simulink model "unit_delay_demo"  (Simulink 6.3)
settings: Solver=ode45  StartTime=0.0  StopTime=10.0  RelTol=1e-3
settings Model: LastModifiedBy=Ms1

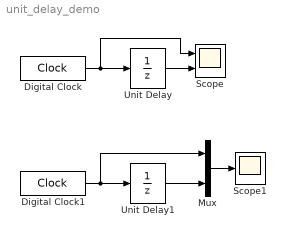
== system unit_delay_demo ==
  Digital Clock : DigitalClock
  Digital Clock1 : DigitalClock
  Mux : Mux  Inputs=2
  Scope : Scope  NumInputPorts=2
      settings: YMin=-5~-5  YMax=5~5
  Scope1 : Scope
  Unit Delay : UnitDelay
  Unit Delay1 : UnitDelay
  wires:
  Digital Clock/1 -> Unit Delay/1, Scope/1
  Unit Delay/1 -> Scope/2
  Digital Clock1/1 -> Unit Delay1/1, Mux/1
  Mux/1 -> Scope1/1
  Unit Delay1/1 -> Mux/2
